simulink library "PrachLib"  (R2022a)
settings: Solver=VariableStepAuto  StartTime=0.0  StopTime=10.0  RelTol=1e-3
values from neighbouring files (symbols this model uses):
  ConfigTable = [16 1 9,20,20,20,20,20,20,20,20,20 0 2 6 2 4 ... (first row only)    [ConfigIndexTable.m]
  NTxAnts = 4    [setup_prach_shortFormat.m]    (also in setup_prach_shortFormat_fftShift.m)
undefined symbols (not defined in the file or in its folder): AdvDSPBChannelOutDisplay, AdvDSPBDMemDisplay, display, dpoly, dspba, dspba_ChannelInVis, dspba_ChannelOutVis, dspba_internal_get_channel_ports, evalAionMaskParam, InstanceNumber, latency, PRACH_regs, prach_short, primtype, UseDontCare, value
libraries: DSPBAPrim x280, DSPBAModelBus x7, DSPBAControl x7, $bdroot x3, DspbAdvFftLibrary x1, DSPBAVectorUtil x1
(part 3 of 4)

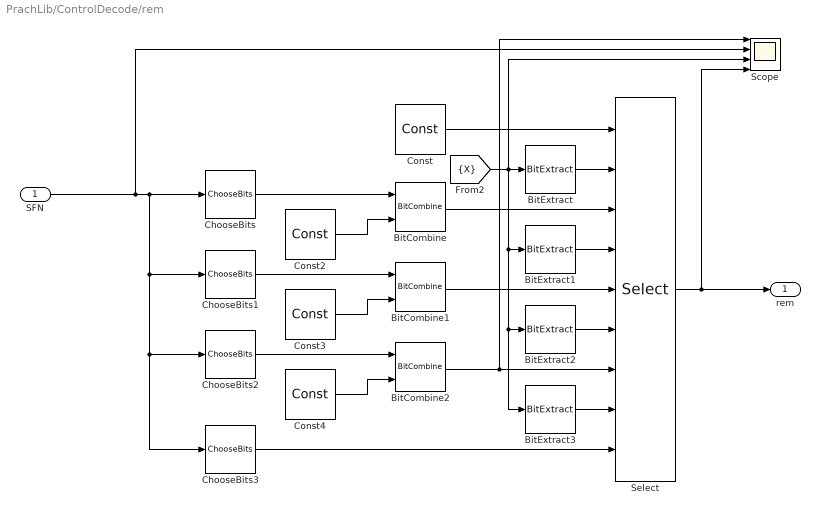
== system PrachLib/ControlDecode/rem ==
  SFN : Inport
  BitCombine : DSPBAPrim/BitCombine  primtype=bitcombine  nInputs=2  nOutputs=1  omode=Inherit via internal rule  otype=sfix(16)  scale=2^-15  rndmethod=Unbiased  factor=1  satmethod=Symmetric  shift_vec=[0 1 2 -1]  value=0  inPortNames=['l'; 'h';]  outPortNames=[' ']  dspbaimage=dspba_prim.svg  text=fprintf('[h,l]');  style=Optimised  visibilities=8+2  version=20211007
  BitCombine1 : DSPBAPrim/BitCombine  primtype=bitcombine  nInputs=2  nOutputs=1  omode=Inherit via internal rule  otype=sfix(16)  scale=2^-15  rndmethod=Unbiased  factor=1  satmethod=Symmetric  shift_vec=[0 1 2 -1]  value=0  inPortNames=['l'; 'h';]  outPortNames=[' ']  dspbaimage=dspba_prim.svg  text=fprintf('[h,l]');  style=Optimised  visibilities=8+2  version=20211007
  BitCombine2 : DSPBAPrim/BitCombine  primtype=bitcombine  nInputs=2  nOutputs=1  omode=Inherit via internal rule  otype=sfix(16)  scale=2^-15  rndmethod=Unbiased  factor=1  satmethod=Symmetric  shift_vec=[0 1 2 -1]  value=0  inPortNames=['l'; 'h';]  outPortNames=[' ']  dspbaimage=dspba_prim.svg  text=fprintf('[h,l]');  style=Optimised  visibilities=8+2  version=20211007
  BitExtract : DSPBAPrim/BitExtract  primtype=bitextract  nInputs=1  nOutputs=1  omode=boolean  otype=ufix(1)  scale=1  rndmethod=Unbiased  factor=1  satmethod=Symmetric  shift_vec=[0 1 2 -1]  value=1  inPortNames=[' '; ' ';]  outPortNames=[' ']  dspbaimage=dspba_prim.svg  text=fprintf('..%d', value);  style=Optimised  visibilities=8+1024  version=20211007
  BitExtract1 : DSPBAPrim/BitExtract  primtype=bitextract  nInputs=1  nOutputs=1  omode=boolean  otype=ufix(1)  scale=1  rndmethod=Unbiased  factor=1  satmethod=Symmetric  shift_vec=[0 1 2 -1]  value=2  inPortNames=[' '; ' ';]  outPortNames=[' ']  dspbaimage=dspba_prim.svg  text=fprintf('..%d', value);  style=Optimised  visibilities=8+1024  version=20211007
  BitExtract2 : DSPBAPrim/BitExtract  primtype=bitextract  nInputs=1  nOutputs=1  omode=boolean  otype=ufix(1)  scale=1  rndmethod=Unbiased  factor=1  satmethod=Symmetric  shift_vec=[0 1 2 -1]  value=3  inPortNames=[' '; ' ';]  outPortNames=[' ']  dspbaimage=dspba_prim.svg  text=fprintf('..%d', value);  style=Optimised  visibilities=8+1024  version=20211007
  BitExtract3 : DSPBAPrim/BitExtract  primtype=bitextract  nInputs=1  nOutputs=1  omode=boolean  otype=ufix(1)  scale=1  rndmethod=Unbiased  factor=1  satmethod=Symmetric  shift_vec=[0 1 2 -1]  value=4  inPortNames=[' '; ' ';]  outPortNames=[' ']  dspbaimage=dspba_prim.svg  text=fprintf('..%d', value);  style=Optimised  visibilities=8+1024  version=20211007
  ChooseBits : DSPBAPrim/ChooseBits  primtype=choosebits  nInputs=1  nOutputs=1  omode=Inherit via internal rule  otype=fixdt(0,1,1)  scale=1  rndmethod=Unbiased  factor=1  satmethod=Symmetric  shift_vec=[0 1 2 -1]  value=[0]  inPortNames=[' '; ' ';]  outPortNames=[' ']  dspbaimage=dspba_prim.svg  text=fprintf('%s',dspba.perm2str(value));  style=Optimised  visibilities=1024  version=20211007
  ChooseBits1 : DSPBAPrim/ChooseBits  primtype=choosebits  nInputs=1  nOutputs=1  omode=Inherit via internal rule  otype=fixdt(0,1,1)  scale=1  rndmethod=Unbiased  factor=1  satmethod=Symmetric  shift_vec=[0 1 2 -1]  value=[0,1]  inPortNames=[' '; ' ';]  outPortNames=[' ']  dspbaimage=dspba_prim.svg  text=fprintf('%s',dspba.perm2str(value));  style=Optimised  visibilities=1024  version=20211007
  ChooseBits2 : DSPBAPrim/ChooseBits  primtype=choosebits  nInputs=1  nOutputs=1  omode=Inherit via internal rule  otype=fixdt(0,1,1)  scale=1  rndmethod=Unbiased  factor=1  satmethod=Symmetric  shift_vec=[0 1 2 -1]  value=[0,1,2]  inPortNames=[' '; ' ';]  outPortNames=[' ']  dspbaimage=dspba_prim.svg  text=fprintf('%s',dspba.perm2str(value));  style=Optimised  visibilities=1024  version=20211007
  ChooseBits3 : DSPBAPrim/ChooseBits  primtype=choosebits  nInputs=1  nOutputs=1  omode=Inherit via internal rule  otype=fixdt(0,1,1)  scale=1  rndmethod=Unbiased  factor=1  satmethod=Symmetric  shift_vec=[0 1 2 -1]  value=[0,1,2,3]  inPortNames=[' '; ' ';]  outPortNames=[' ']  dspbaimage=dspba_prim.svg  text=fprintf('%s',dspba.perm2str(value));  style=Optimised  visibilities=1024  version=20211007
  Const : DSPBAPrim/Const  primtype=const  nInputs=0  nOutputs=1  omode=Specify via dialog  otype=ufix(4)  scale=1  rndmethod=Unbiased  factor=1  satmethod=Symmetric  shift_vec=[0 1 2 -1]  value=0  inPortNames=['+'; '+';]  outPortNames=[' ']  dspbaimage=dspba_prim.svg  text=fprintf('%s', num2str(value));  style=Optimised  visibilities=8 + 1024  floatPrecision=float32_m23  warnSaturation=on  version=20211007  SampleTime=inf
  Const2 : DSPBAPrim/Const  primtype=const  nInputs=0  nOutputs=1  omode=Specify via dialog  otype=ufix(3)  scale=1  rndmethod=Unbiased  factor=1  satmethod=Symmetric  shift_vec=[0 1 2 -1]  value=0  inPortNames=['+'; '+';]  outPortNames=[' ']  dspbaimage=dspba_prim.svg  text=fprintf('%s', num2str(value));  style=Optimised  visibilities=8 + 1024  floatPrecision=float32_m23  warnSaturation=on  version=20211007  SampleTime=inf
  Const3 : DSPBAPrim/Const  primtype=const  nInputs=0  nOutputs=1  omode=Specify via dialog  otype=ufix(2)  scale=1  rndmethod=Unbiased  factor=1  satmethod=Symmetric  shift_vec=[0 1 2 -1]  value=0  inPortNames=['+'; '+';]  outPortNames=[' ']  dspbaimage=dspba_prim.svg  text=fprintf('%s', num2str(value));  style=Optimised  visibilities=8 + 1024  floatPrecision=float32_m23  warnSaturation=on  version=20211007  SampleTime=inf
  Const4 : DSPBAPrim/Const  primtype=const  nInputs=0  nOutputs=1  omode=Specify via dialog  otype=ufix(1)  scale=1  rndmethod=Unbiased  factor=1  satmethod=Symmetric  shift_vec=[0 1 2 -1]  value=0  inPortNames=['+'; '+';]  outPortNames=[' ']  dspbaimage=dspba_prim.svg  text=fprintf('%s', num2str(value));  style=Optimised  visibilities=8 + 1024  floatPrecision=float32_m23  warnSaturation=on  version=20211007  SampleTime=inf
  Scope : Scope  NumInputPorts=4
  Select : DSPBAPrim/Select  primtype=select  nInputs=str2num(get_param(gcb,'value'))*2+1  nOutputs=1  omode=Inherit via internal rule  otype=sfix(16)  scale=2^-15  rndmethod=Unbiased  factor=1  satmethod=Symmetric  shift_vec=[0 1 2 -1]  value=4  inPortNames=['d'; '0'; 'a'; '1'; 'b'; '2'; 'c'; '3'; 'd'; '4'; 'e'; '5'; 'f'; '6'; 'g'; '7'; 'h'; '8'; 'i'; '9'; 'j']  outPortNames=[' ']  dspbaimage=dspba_prim_tall.svg  text=fprintf('%s', primtype);  style=Optimised  visibilities=8 + 1024  version=20211007
  rem : Outport
  wires:
  BitCombine2/1 -> Select/7, Scope/1
  SFN/1 -> ChooseBits/1, ChooseBits1/1, ChooseBits2/1, ChooseBits3/1, Scope/2
  [X] -> BitExtract/1, BitExtract3/1, BitExtract2/1, BitExtract1/1, Scope/3
  ChooseBits1/1 -> BitCombine1/1
  ChooseBits2/1 -> BitCombine2/1
  BitExtract1/1 -> Select/4
  ChooseBits/1 -> BitCombine/1
  BitCombine/1 -> Select/3
  Const2/1 -> BitCombine/2
  Const3/1 -> BitCombine1/2
  BitExtract/1 -> Select/2
  BitExtract3/1 -> Select/8
  Select/1 -> rem/1, Scope/4
  BitCombine1/1 -> Select/5
  Const4/1 -> BitCombine2/2
  BitExtract2/1 -> Select/6
  ChooseBits3/1 -> Select/9
  Const/1 -> Select/1

== system PrachLib/PRACH_CC/ScaleAndSelect ==
  vin : Inport
  chin : Inport  Port=2
  FFTSize : Inport  Port=3
  d : Inport  Port=4
  BWby10 : Inport  Port=5
  And1 : DSPBAPrim/And  primtype=and  nInputs=2  nOutputs=1  omode=Inherit via internal rule  otype=sfix(16)  scale=2^-15  rndmethod=Unbiased  factor=1  satmethod=Symmetric  shift_vec=[0 1 2 -1]  value=0  inPortNames=[' '; ' '; ' '; ' '; ' '; ' '; ' '; ' '; ' '; ' '; ' '; ' '; ' '; ' '; ' '; ' '; ]  outPortNames=[' ']  dspbaimage=dspba_prim.svg  text=fprintf('&');  style=Optimised  visibilities=8+2  version=20211007
  ChannelIn : DSPBAPrim/ChannelIn  primtype=channelin  nInputs=dspba_internal_get_channel_ports(gcb)  nOutputs=dspba_internal_get_channel_ports(gcb)  omode=Inherit via internal rule  otype=sfix(16)  scale=2^-15  rndmethod=Unbiased  factor=1  satmethod=Symmetric  shift_vec=[0 1 2 -1]  value=3  inPortNames=['v'; 'c'; '0'; '1'; '2'; '3'; '4'; '5'; '6'; '7'; '8'; '9'; 'A'; 'B'; 'D'; 'E'; 'F'; 'G'; 'H'; 'I'; 'J'; 'K'; 'L'; 'M'; 'N'; 'O'; 'P'; 'Q'; 'R'; 'S'; 'T'; 'U'; 'W'; 'X'; 'Y'; 'Z']  outPortNames=['v'; 'c'; '0'; '1'; '2'; '3'; '4'; '5'; '6'; '7'; '8'; '9'; 'A'; 'B'; 'D'; 'E'; 'F'; 'G'; 'H'; 'I'; 'J'; 'K'; 'L'; 'M'; 'N'; 'O'; 'P'; 'Q'; 'R'; 'S'; 'T'; 'U'; 'W'; 'X'; 'Y'; 'Z']  dspbaimage=dspba_prim_channel_tall.svg  text=fprintf('In');  style=Optimised  dataSignals=3  foldingEnabled=off  channels=1  sampleRate=200  packetBeginPresent=off  packetBeginEnabled=off  visibilities=dspba_ChannelInVis(gcb)  latencyCorrection=0  scheduleOrigin=off  version=20211214
  ChannelOut : DSPBAPrim/ChannelOut  primtype=channelout  nInputs=dspba_internal_get_channel_ports(gcb)  nOutputs=dspba_internal_get_channel_ports(gcb)  omode=Inherit via internal rule  otype=sfix(16)  scale=2^-15  rndmethod=Unbiased  factor=1  satmethod=Symmetric  shift_vec=[0 1 2 -1]  value=3  inPortNames=['v'; 'c'; '0'; '1'; '2'; '3'; '4'; '5'; '6'; '7'; '8'; '9'; 'A'; 'B'; 'D'; 'E'; 'F'; 'G'; 'H'; 'I'; 'J'; 'K'; 'L'; 'M'; 'N'; 'O'; 'P'; 'Q'; 'R'; 'S'; 'T'; 'U'; 'W'; 'X'; 'Y'; 'Z']  outPortNames=['v'; 'c'; '0'; '1'; '2'; '3'; '4'; '5'; '6'; '7'; '8'; '9'; 'A'; 'B'; 'D'; 'E'; 'F'; 'G'; 'H'; 'I'; 'J'; 'K'; 'L'; 'M'; 'N'; 'O'; 'P'; 'Q'; 'R'; 'S'; 'T'; 'U'; 'W'; 'X'; 'Y'; 'Z']  dspbaimage=dspba_prim_channel_tall.svg  text=fprintf('Out%s', AdvDSPBChannelOutDisplay(latency));  style=Optimised  dataSignals=3  foldingEnabled=off  channels=1  sampleRate=200  packetBeginPresent=off  packetBeginEnabled=off  visibilities=dspba_ChannelOutVis(gcb)  latency=0  latencyCorrection=0  version=20211214
  IndexCounter : Subsystem
  ScaleOutputAndCheck : Subsystem
      mask Display:
      | color('w');image('dspba_prim.jpg');
      | fprintf('*2^PRACH_fft_scale');
      | port_label('input',1,'din');
      | port_label('output',1,'dout');
  Sub : DSPBAPrim/Sub  primtype=sub  nInputs=2  nOutputs=1  omode=Inherit via internal rule with word growth  otype=sfix(16)  scale=2^-15  rndmethod=Unbiased  factor=1  satmethod=Symmetric  shift_vec=[0 1 2 -1]  value=0  inPortNames=['+'; '-';]  outPortNames=[' ']  dspbaimage=dspba_prim.svg  text=fprintf('-');  style=Optimised  visibilities=8+2^17+2^18  floatRounding=correct  advOptions=[]  version=20211007
  SynthesisInfo : DSPBAPrim/SynthesisInfo  primtype=synthinfo  nInputs=0  nOutputs=0  omode=Inherit via internal rule  otype=sfix(16)  scale=2^-15  rndmethod=Truncate  factor=1  satmethod=Symmetric  shift_vec=[0 1 2 -1]  value=99  inPortNames=[' '; ' ';]  outPortNames=[' ']  dspbaimage=dspba_prim_ctrl.jpg  text=fprintf('Style=%s', style);  style=Scheduled  visibilities=32768  constraintPair=None  constraintRelation=>  constraintLimit=6  modelRefSign=+  modelRef=''  showSchedule=off  simulationMode=Use Global Value  resetMinimization=Conditional - On for ChannelIn/Out only  version=20220106
  gen_139_valids : Subsystem
  qv : Outport  VectorParamsAs1DForOutWhenUnconnected=off
  qch : Outport  Port=2  VectorParamsAs1DForOutWhenUnconnected=off
  q : Outport  Port=3  VectorParamsAs1DForOutWhenUnconnected=off
  qv139 : Outport  Port=4  VectorParamsAs1DForOutWhenUnconnected=off
  FreqBinIdx : Outport  Port=5  VectorParamsAs1DForOutWhenUnconnected=off
  wires:
  ChannelOut/1 -> qv/1
  ChannelOut/2 -> qch/1
  ChannelIn/1 -> And1/1, ChannelOut/1, IndexCounter/1(v)
  ChannelIn/2 -> ChannelOut/2
  vin/1 -> ChannelIn/1
  chin/1 -> ChannelIn/2
  ChannelOut/3 -> q/1
  ChannelOut/4 -> qv139/1
  FFTSize/1 -> ChannelIn/3
  d/1 -> ChannelIn/4
  ChannelIn/4 -> ScaleOutputAndCheck/1(din)
  ChannelOut/5 -> FreqBinIdx/1
  BWby10/1 -> ChannelIn/5
  And1/1 -> ChannelOut/4
  IndexCounter/1(index) -> Sub/1, gen_139_valids/1(Index)
  gen_139_valids/1(v139) -> And1/2
  ChannelIn/5 -> gen_139_valids/3(BWby10)
  ChannelIn/3 -> gen_139_valids/2(FFTSize), IndexCounter/2(FFTSize)
  gen_139_valids/2(startSymFD) -> Sub/2
  Sub/1 -> ChannelOut/5
  ScaleOutputAndCheck/1(dout) -> ChannelOut/3

== system PrachLib/PRACH_CC/VFFT ==
  note: Bit-accurate simulation used
  note: Each block of 2^N samples should use the same channel
      | and starts arriving on the output after 2^N-1 cycles.
      |
      | So we latch the channel number and size on
      |  the last valid input of each block.
  v : Inport
  c : Inport  Port=2
  size : Inport  Port=3
  d : Inport  Port=4
  BWby10 : Inport  Port=5
  ChannelIn : DSPBAPrim/ChannelIn  primtype=channelin  nInputs=dspba_internal_get_channel_ports(gcb)  nOutputs=dspba_internal_get_channel_ports(gcb)  omode=Inherit via internal rule  otype=sfix(16)  scale=2^-15  rndmethod=Unbiased  factor=1  satmethod=Symmetric  shift_vec=[0 1 2 -1]  value=3  inPortNames=['v'; 'c'; '0'; '1'; '2'; '3'; '4'; '5'; '6'; '7'; '8'; '9'; 'a'; 'b']  outPortNames=['v'; 'c'; '0'; '1'; '2'; '3'; '4'; '5'; '6'; '7'; '8'; '9'; 'a'; 'b']  dspbaimage=dspba_prim_channel_tall.svg  text=fprintf('In');  style=Optimised  dataSignals=3  foldingEnabled=off  channels=1  sampleRate=200  packetBeginPresent=off  packetBeginEnabled=off  visibilities=dspba_ChannelInVis(gcb)  latencyCorrection=0  scheduleOrigin=on  version=20211214
  ChannelOut1 : DSPBAPrim/ChannelOut  primtype=channelout  nInputs=dspba_internal_get_channel_ports(gcb)  nOutputs=dspba_internal_get_channel_ports(gcb)  omode=Inherit via internal rule  otype=sfix(16)  scale=2^-15  rndmethod=Unbiased  factor=1  satmethod=Symmetric  shift_vec=[0 1 2 -1]  value=3  inPortNames=['v'; 'c'; '0'; '1'; '2'; '3'; '4'; '5'; '6'; '7'; '8'; '9']  outPortNames=['v'; 'c'; '0'; '1'; '2'; '3'; '4'; '5'; '6'; '7'; '8'; '9']  dspbaimage=dspba_prim_channel_tall.svg  text=fprintf('Out');  style=Optimised  dataSignals=3  foldingEnabled=off  channels=1  sampleRate=200  packetBeginPresent=off  packetBeginEnabled=off  visibilities=dspba_ChannelOutVis(gcb)  latency=0  latencyCorrection=0  version=20211214
  SynthesisInfo : DSPBAPrim/SynthesisInfo  primtype=synthinfo  nInputs=0  nOutputs=0  omode=Inherit via internal rule  otype=sfix(16)  scale=2^-15  rndmethod=Truncate  factor=1  satmethod=Symmetric  shift_vec=[0 1 2 -1]  value=99  inPortNames=[' '; ' ';]  outPortNames=[' ']  dspbaimage=dspba_prim_ctrl.jpg  text=fprintf('Style=%s', style);  style=Scheduled  visibilities=32768  constraintPair=None  constraintRelation=>  constraintLimit=2  modelRefSign=+  modelRef=''  showSchedule=off  simulationMode=Bit Accurate  resetMinimization=Conditional - On for ChannelIn/Out only  version=20220106
  VFFT_Light : DspbAdvFftLibrary/Common/VFFT_Light  IFFT=IFFT  subchannels=subchannels  br_in=br_in  maxSize=maxSize  minSize=minSize  in_type=in_type  type_strings=type_strings  faithful=faithful  wirecount=1
  latch_0L : DSPBAControl/latch_0L
  latch_0L1 : DSPBAControl/latch_0L
  latch_0L2 : DSPBAControl/latch_0L
  qv : Outport
  qc : Outport  Port=2
  qsize : Outport  Port=3
  q : Outport  Port=4
  qBWby10 : Outport  Port=5
  wires:
  VFFT_Light/2 -> ChannelOut1/4
  latch_0L1/1 -> ChannelOut1/3
  ChannelOut1/3 -> qsize/1
  ChannelOut1/4 -> q/1
  ChannelIn/4 -> VFFT_Light/3
  ChannelIn/3 -> VFFT_Light/2, latch_0L1/2
  d/1 -> ChannelIn/4
  size/1 -> ChannelIn/3
  v/1 -> ChannelIn/1
  c/1 -> ChannelIn/2
  latch_0L/1 -> ChannelOut1/2
  ChannelIn/2 -> latch_0L/2
  ChannelOut1/1 -> qv/1
  ChannelOut1/2 -> qc/1
  VFFT_Light/1 -> ChannelOut1/1
  ChannelIn/1 -> VFFT_Light/1
  VFFT_Light/3 -> latch_0L2/1, latch_0L1/1, latch_0L/1
  BWby10/1 -> ChannelIn/5
  ChannelIn/5 -> latch_0L2/2
  latch_0L2/1 -> ChannelOut1/5
  ChannelOut1/5 -> qBWby10/1

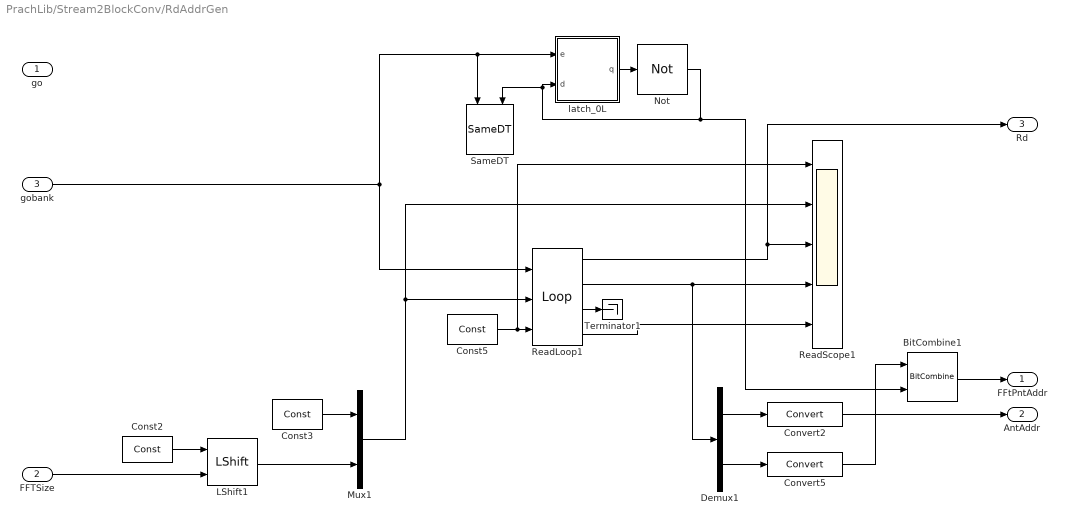
== system PrachLib/Stream2BlockConv/RdAddrGen ==
  go : Inport
  FFTSize : Inport  Port=2
  gobank : Inport  Port=3
  BitCombine1 : DSPBAPrim/BitCombine  primtype=bitcombine  nInputs=2  nOutputs=1  omode=Inherit via internal rule  otype=sfix(16)  scale=2^-15  rndmethod=Unbiased  factor=1  satmethod=Symmetric  shift_vec=[0 1 2 -1]  value=0  inPortNames=['l'; 'h';]  outPortNames=[' ']  dspbaimage=dspba_prim.svg  text=fprintf('[h,l]');  style=Optimised  visibilities=8+2  version=20211007
  Const2 : DSPBAPrim/Const  primtype=const  nInputs=0  nOutputs=1  omode=Inherit via internal rule  otype=sfix(16)  scale=2^-15  rndmethod=Unbiased  factor=1  satmethod=Symmetric  shift_vec=[0 1 2 -1]  value=1  inPortNames=['+'; '+';]  outPortNames=[' ']  dspbaimage=dspba_prim.svg  text=fprintf('%s', num2str(value));  style=Optimised  visibilities=8 + 1024  floatPrecision=float32_m23  warnSaturation=on  version=20211007  SampleTime=inf
  Const3 : DSPBAPrim/Const  primtype=const  nInputs=0  nOutputs=1  omode=Inherit via back propagation  otype=sfix(16)  scale=2^-15  rndmethod=Unbiased  factor=1  satmethod=Symmetric  shift_vec=[0 1 2 -1]  value=NAnts  inPortNames=['+'; '+';]  outPortNames=[' ']  dspbaimage=dspba_prim.svg  text=fprintf('%s', num2str(value));  style=Optimised  visibilities=8 + 1024  floatPrecision=float32_m23  warnSaturation=on  version=20211007  SampleTime=inf
  Const5 : DSPBAPrim/Const  primtype=const  nInputs=0  nOutputs=1  omode=boolean  otype=sfix(16)  scale=2^-15  rndmethod=Unbiased  factor=1  satmethod=Symmetric  shift_vec=[0 1 2 -1]  value=1  inPortNames=['+'; '+';]  outPortNames=[' ']  dspbaimage=dspba_prim.svg  text=fprintf('%s', num2str(value));  style=Optimised  visibilities=8 + 1024  floatPrecision=float32_m23  warnSaturation=on  version=20211007  SampleTime=inf
  Convert2 : DSPBAPrim/Convert  primtype=convert  nInputs=1  nOutputs=1  omode=Specify via dialog  otype=ufix(ceil(log2(NAnts)))  scale=1  rndmethod=Truncate  factor=1  satmethod=None  shift_vec=[0 1 2 -1]  value=round([0:255]/17)  inPortNames=[' '; ' ';]  outPortNames=[' '; 'c']  dspbaimage=dspba_prim_wide.svg  text=fprintf('convert');  style=Optimised  visibilities=8+64+256+2^17  clipdetect=off  floatPrecision=float32_m23  advOptions=[]  version=20211007
  Convert5 : DSPBAPrim/Convert  primtype=convert  nInputs=1  nOutputs=1  omode=Specify via dialog  otype=ufix(ceil(log2(NFftMax)))  scale=1  rndmethod=Truncate  factor=1  satmethod=None  shift_vec=[0 1 2 -1]  value=round([0:255]/17)  inPortNames=[' '; ' ';]  outPortNames=[' '; 'c']  dspbaimage=dspba_prim_wide.svg  text=fprintf('convert');  style=Optimised  visibilities=8+64+256+2^17  clipdetect=off  floatPrecision=float32_m23  advOptions=[]  version=20211007
  Demux1 : Demux  Outputs=2
  LShift1 : DSPBAPrim/LShift  primtype=lshift  nInputs=2  nOutputs=1  omode=Specify via dialog  otype=ufix(log2(NFftMax)+1)  scale=1  rndmethod=Unbiased  factor=1  satmethod=Symmetric  shift_vec=[0 1 2 -1]  value=0  inPortNames=['a'; 'b';]  outPortNames=[' ']  dspbaimage=dspba_prim.svg  text=fprintf('a << b');  style=Optimised  visibilities=8  version=20211007
  Mux1 : Mux  Inputs=2
  Not : DSPBAPrim/Not  primtype=not  nInputs=1  nOutputs=1  omode=Inherit via internal rule  otype=sfix(16)  scale=2^-15  rndmethod=Unbiased  factor=1  satmethod=Symmetric  shift_vec=[0 1 2 -1]  value=0  inPortNames=[' '; ' ';]  outPortNames=[' ']  dspbaimage=dspba_prim.svg  text=fprintf('~');  style=Optimised  visibilities=8  version=20211007
  ReadLoop1 : DSPBAPrim/Loop  primtype=loop  nInputs=3  nOutputs=4  omode=Inherit via internal rule  otype=sfix(16)  scale=2^-15  rndmethod=Unbiased  factor=1  satmethod=Symmetric  shift_vec=[0 1 2 -1]  value=[zeros(16, 1)]  inPortNames=['g'; 'c'; 'e']  outPortNames=['v'; 'q'; 'f'; 'l']  dspbaimage=dspba_prim_tall.svg  text=fprintf('loop');  style=Optimised  visibilities=0  version=20211007
  ReadScope1 : Scope  NumInputPorts=5
  SameDT : DSPBAControl/SameDT
  Terminator1 : Terminator
  latch_0L : Subsystem  AncestorBlock=DSPBAControl/latch_0L
      mask help: The latch_0 block enable signal has an immediate effect on the output. While the enable is high,the data passes straight through.When the enable goes low, the latch_0 block outputs and holds the data input from the previous cycle.
      mask Help: helpview(dspba.GetHelp('latch_0L'));
      mask Display:
      | color('w');
      | image('dspba_prim_masked.png');
      | fprintf('0L\nlatch');
      | port_label('input',1,'e');
      | port_label('input',2,'d');
      | port_label('output',1,'q');
  FFtPntAddr : Outport
  AntAddr : Outport  Port=2
  Rd : Outport  Port=3
  wires:
  latch_0L/1(q) -> Not/1
  BitCombine1/1 -> FFtPntAddr/1
  gobank/1 -> ReadLoop1/1, latch_0L/1(e), SameDT/1
  Not/1 -> BitCombine1/2, SameDT/2, latch_0L/2(d)
  Demux1/2 -> Convert5/1
  Demux1/1 -> Convert2/1
  Const2/1 -> LShift1/1
  Mux1/1 -> ReadLoop1/2, ReadScope1/2
  Const5/1 -> ReadScope1/1, ReadLoop1/3
  FFTSize/1 -> LShift1/2
  ReadLoop1/2 -> Demux1/1, ReadScope1/4
  ReadLoop1/1 -> ReadScope1/3, Rd/1
  Const3/1 -> Mux1/1
  ReadLoop1/3 -> Terminator1/1
  Convert5/1 -> BitCombine1/1
  LShift1/1 -> Mux1/2
  ReadLoop1/4 -> ReadScope1/5
  Convert2/1 -> AntAddr/1

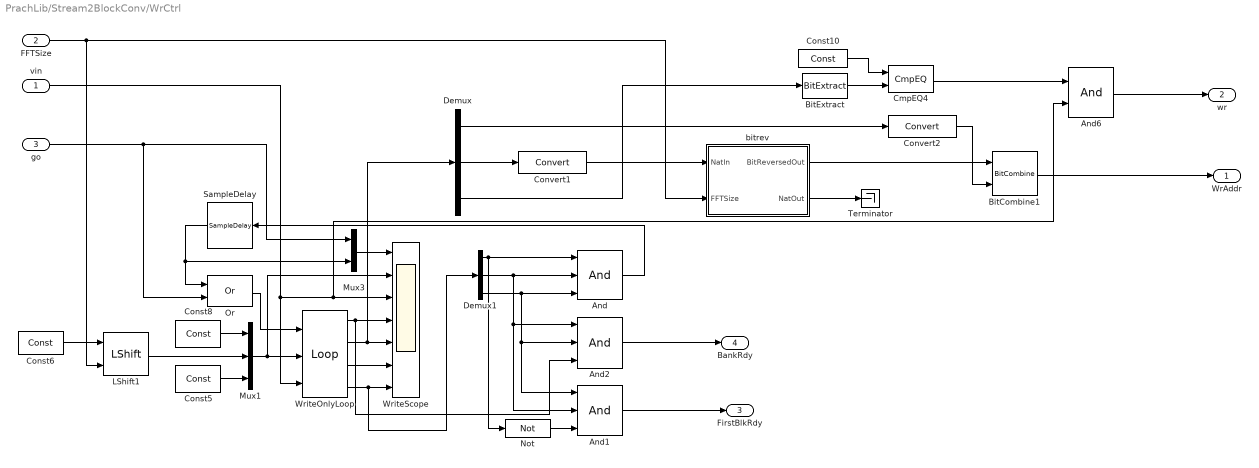
== system PrachLib/Stream2BlockConv/WrCtrl ==
  vin : Inport
  FFTSize : Inport  Port=2
  go : Inport  Port=3
  And : DSPBAPrim/And  primtype=and  nInputs=3  nOutputs=1  omode=Inherit via internal rule  otype=sfix(16)  scale=2^-15  rndmethod=Unbiased  factor=1  satmethod=Symmetric  shift_vec=[0 1 2 -1]  value=0  inPortNames=[' '; ' '; ' '; ' '; ' '; ' '; ' '; ' '; ' '; ' '; ' '; ' '; ' '; ' '; ' '; ' '; ]  outPortNames=[' ']  dspbaimage=dspba_prim.svg  text=fprintf('&');  style=Optimised  visibilities=8+2  version=20211007
  And1 : DSPBAPrim/And  primtype=and  nInputs=3  nOutputs=1  omode=Inherit via internal rule  otype=sfix(16)  scale=2^-15  rndmethod=Unbiased  factor=1  satmethod=Symmetric  shift_vec=[0 1 2 -1]  value=0  inPortNames=[' '; ' '; ' '; ' '; ' '; ' '; ' '; ' '; ' '; ' '; ' '; ' '; ' '; ' '; ' '; ' '; ]  outPortNames=[' ']  dspbaimage=dspba_prim.svg  text=fprintf('&');  style=Optimised  visibilities=8+2  version=20211007
  And2 : DSPBAPrim/And  primtype=and  nInputs=3  nOutputs=1  omode=Inherit via internal rule  otype=sfix(16)  scale=2^-15  rndmethod=Unbiased  factor=1  satmethod=Symmetric  shift_vec=[0 1 2 -1]  value=0  inPortNames=[' '; ' '; ' '; ' '; ' '; ' '; ' '; ' '; ' '; ' '; ' '; ' '; ' '; ' '; ' '; ' '; ]  outPortNames=[' ']  dspbaimage=dspba_prim.svg  text=fprintf('&');  style=Optimised  visibilities=8+2  version=20211007
  And6 : DSPBAPrim/And  primtype=and  nInputs=2  nOutputs=1  omode=Inherit via internal rule  otype=sfix(16)  scale=2^-15  rndmethod=Unbiased  factor=1  satmethod=Symmetric  shift_vec=[0 1 2 -1]  value=0  inPortNames=[' '; ' '; ' '; ' '; ' '; ' '; ' '; ' '; ' '; ' '; ' '; ' '; ' '; ' '; ' '; ' '; ]  outPortNames=[' ']  dspbaimage=dspba_prim.svg  text=fprintf('&');  style=Optimised  visibilities=8+2  version=20211007
  BitCombine1 : DSPBAPrim/BitCombine  primtype=bitcombine  nInputs=2  nOutputs=1  omode=Inherit via internal rule  otype=sfix(16)  scale=2^-15  rndmethod=Unbiased  factor=1  satmethod=Symmetric  shift_vec=[0 1 2 -1]  value=0  inPortNames=['l'; 'h';]  outPortNames=[' ']  dspbaimage=dspba_prim.svg  text=fprintf('[h,l]');  style=Optimised  visibilities=8+2  version=20211007
  BitExtract : DSPBAPrim/BitExtract  primtype=bitextract  nInputs=1  nOutputs=1  omode=Specify via dialog  otype=ufix(ceil(log2(NTxAnts)))  scale=1  rndmethod=Unbiased  factor=1  satmethod=Symmetric  shift_vec=[0 1 2 -1]  value=0  inPortNames=[' '; ' ';]  outPortNames=[' ']  dspbaimage=dspba_prim.svg  text=fprintf('..%d', value);  style=Optimised  visibilities=8+1024  version=20211007
  CmpEQ4 : DSPBAPrim/CmpEQ  primtype=cmpeq  nInputs=2  nOutputs=1  omode=boolean  otype=sfix(16)  scale=2^-15  rndmethod=Unbiased  factor=1  satmethod=Symmetric  shift_vec=[0 1 2 -1]  value=0  inPortNames=[' '; ' ';]  outPortNames=[' ']  dspbaimage=dspba_prim.svg  text=fprintf('==');  style=Optimised  visibilities=0  advOptions=[]  version=20211007
  Const10 : DSPBAPrim/Const  primtype=const  nInputs=0  nOutputs=1  omode=Inherit via internal rule  otype=sfix(16)  scale=2^-15  rndmethod=Unbiased  factor=1  satmethod=Symmetric  shift_vec=[0 1 2 -1]  value=0:(NTxAnts-1)  inPortNames=['+'; '+';]  outPortNames=[' ']  dspbaimage=dspba_prim.svg  text=fprintf('%s', num2str(value));  style=Optimised  visibilities=8 + 1024  floatPrecision=float32_m23  warnSaturation=on  version=20211007  SampleTime=inf
  Const5 : DSPBAPrim/Const  primtype=const  nInputs=0  nOutputs=1  omode=Inherit via back propagation  otype=sfix(16)  scale=2^-15  rndmethod=Unbiased  factor=1  satmethod=Symmetric  shift_vec=[0 1 2 -1]  value=NAnts  inPortNames=['+'; '+';]  outPortNames=[' ']  dspbaimage=dspba_prim.svg  text=fprintf('%s', num2str(value));  style=Optimised  visibilities=8 + 1024  floatPrecision=float32_m23  warnSaturation=on  version=20211007  SampleTime=inf
  Const6 : DSPBAPrim/Const  primtype=const  nInputs=0  nOutputs=1  omode=Inherit via internal rule  otype=sfix(16)  scale=2^-15  rndmethod=Unbiased  factor=1  satmethod=Symmetric  shift_vec=[0 1 2 -1]  value=1  inPortNames=['+'; '+';]  outPortNames=[' ']  dspbaimage=dspba_prim.svg  text=fprintf('%s', num2str(value));  style=Optimised  visibilities=8 + 1024  floatPrecision=float32_m23  warnSaturation=on  version=20211007  SampleTime=inf
  Const8 : DSPBAPrim/Const  primtype=const  nInputs=0  nOutputs=1  omode=Inherit via back propagation  otype=sfix(16)  scale=2^-15  rndmethod=Unbiased  factor=1  satmethod=Symmetric  shift_vec=[0 1 2 -1]  value=2  inPortNames=['+'; '+';]  outPortNames=[' ']  dspbaimage=dspba_prim.svg  text=fprintf('%s', num2str(value));  style=Optimised  visibilities=8 + 1024  floatPrecision=float32_m23  warnSaturation=on  version=20211007  SampleTime=inf
  Convert1 : DSPBAPrim/Convert  primtype=convert  nInputs=1  nOutputs=1  omode=Specify via dialog  otype=ufix(ceil(log2(NFftMax)))  scale=1  rndmethod=Truncate  factor=1  satmethod=None  shift_vec=[0 1 2 -1]  value=round([0:255]/17)  inPortNames=[' '; ' ';]  outPortNames=[' '; 'c']  dspbaimage=dspba_prim_wide.svg  text=fprintf('convert');  style=Optimised  visibilities=8+64+256+2^17  clipdetect=off  floatPrecision=float32_m23  advOptions=[]  version=20211007
  Convert2 : DSPBAPrim/Convert  primtype=convert  nInputs=1  nOutputs=1  omode=Specify via dialog  otype=ufix(1)  scale=1  rndmethod=Truncate  factor=1  satmethod=None  shift_vec=[0 1 2 -1]  value=round([0:255]/17)  inPortNames=[' '; ' ';]  outPortNames=[' '; 'c']  dspbaimage=dspba_prim_wide.svg  text=fprintf('convert');  style=Optimised  visibilities=8+64+256+2^17  clipdetect=off  floatPrecision=float32_m23  advOptions=[]  version=20211007
  Demux : Demux  Outputs=3
  Demux1 : Demux  Outputs=3
  LShift1 : DSPBAPrim/LShift  primtype=lshift  nInputs=2  nOutputs=1  omode=Specify via dialog  otype=ufix(log2(NFftMax)+1)  scale=1  rndmethod=Unbiased  factor=1  satmethod=Symmetric  shift_vec=[0 1 2 -1]  value=0  inPortNames=['a'; 'b';]  outPortNames=[' ']  dspbaimage=dspba_prim.svg  text=fprintf('a << b');  style=Optimised  visibilities=8  version=20211007
  Mux1 : Mux  Inputs=3
  Mux3 : Mux  Inputs=2
  Not : DSPBAPrim/Not  primtype=not  nInputs=1  nOutputs=1  omode=Inherit via internal rule  otype=sfix(16)  scale=2^-15  rndmethod=Unbiased  factor=1  satmethod=Symmetric  shift_vec=[0 1 2 -1]  value=0  inPortNames=[' '; ' ';]  outPortNames=[' ']  dspbaimage=dspba_prim.svg  text=fprintf('~');  style=Optimised  visibilities=8  version=20211007
  Or : DSPBAPrim/Or  primtype=or  nInputs=2  nOutputs=1  omode=Inherit via internal rule  otype=sfix(16)  scale=2^-15  rndmethod=Unbiased  factor=1  satmethod=Symmetric  shift_vec=[0 1 2 -1]  value=0  inPortNames=[' '; ' '; ' '; ' '; ' '; ' '; ' '; ' '; ' '; ' '; ' '; ' '; ' '; ' '; ' '; ' '; ]  outPortNames=[' ']  dspbaimage=dspba_prim.svg  text=fprintf('|');  style=Optimised  visibilities=8+2  version=20211007
  SampleDelay : DSPBAPrim/SampleDelay  primtype=sampdelay  nInputs=1  nOutputs=1  omode=Inherit via internal rule  otype=sfix(16)  scale=2^-15  rndmethod=Unbiased  factor=1  satmethod=Symmetric  shift_vec=[0 1 2 -1]  floatPrecision=float32_m23  value=1  inPortNames=[' '; ' ';]  outPortNames=[' ']  dspbaimage=dspba_prim.svg  text=dpoly(1, eye(1,value+1), 'z')  style=Optimised  visibilities=8 + 1024 + 2^17 + 2^18  flexible=off  slackgroup=0  augmented=0  version=20211007  advOptions=[]
  Terminator : Terminator
  WriteOnlyLoop : DSPBAPrim/Loop  primtype=loop  nInputs=3  nOutputs=4  omode=Inherit via internal rule  otype=sfix(16)  scale=2^-15  rndmethod=Unbiased  factor=1  satmethod=Symmetric  shift_vec=[0 1 2 -1]  value=[zeros(16, 1)]  inPortNames=['g'; 'c'; 'e']  outPortNames=['v'; 'q'; 'f'; 'l']  dspbaimage=dspba_prim_tall.svg  text=fprintf('loop');  style=Optimised  visibilities=0  version=20211007
  WriteScope : Scope  NumInputPorts=7
  bitrev : Subsystem  mask{NFftMax=NFftMax}
      mask prompts: NFftMax "Maximum FFT size"
  WrAddr : Outport
  wr : Outport  Port=2
  FirstBlkRdy : Outport  Port=3
  BankRdy : Outport  Port=4
  wires:
  And2/1 -> BankRdy/1
  bitrev/1(BitReversedOut) -> BitCombine1/1
  bitrev/2(NatOut) -> Terminator/1
  And6/1 -> wr/1
  Convert2/1 -> BitCombine1/2
  Mux3/1 -> WriteScope/1
  Const10/1 -> CmpEQ4/1
  Convert1/1 -> bitrev/1(NatIn)
  And/1 -> SampleDelay/1
  LShift1/1 -> Mux1/2
  Const6/1 -> LShift1/1
  BitCombine1/1 -> WrAddr/1
  vin/1 -> WriteScope/3, And6/2, WriteOnlyLoop/3
  Demux1/3 -> And/3, And2/2, And1/1
  WriteOnlyLoop/4 -> Demux1/1, WriteScope/7
  And1/1 -> FirstBlkRdy/1
  FFTSize/1 -> bitrev/2(FFTSize), LShift1/2
  Or/1 -> WriteOnlyLoop/1
  WriteOnlyLoop/3 -> WriteScope/6
  SampleDelay/1 -> Mux3/2, Or/1
  Demux1/2 -> And/2, And2/1, And1/2
  Demux/3 -> BitExtract/1
  Demux/2 -> Convert1/1
  Demux1/1 -> Not/1, And/1
  Not/1 -> And1/3
  Demux/1 -> Convert2/1
  BitExtract/1 -> CmpEQ4/2
  Mux1/1 -> WriteScope/2, WriteOnlyLoop/2
  WriteOnlyLoop/1 -> WriteScope/4, And2/3
  WriteOnlyLoop/2 -> WriteScope/5, Demux/1
  Const5/1 -> Mux1/3
  go/1 -> Or/2, Mux3/1
  Const8/1 -> Mux1/1
  CmpEQ4/1 -> And6/1

== system PrachLib/PRACH_CC/ScaleAndSelect/IndexCounter ==
  v : Inport
  FFTSize : Inport  Port=2
  And : DSPBAPrim/And  primtype=and  nInputs=2  nOutputs=1  omode=Inherit via internal rule  otype=sfix(16)  scale=2^-15  rndmethod=Unbiased  factor=1  satmethod=Symmetric  shift_vec=[0 1 2 -1]  value=0  inPortNames=[' '; ' '; ' '; ' '; ' '; ' '; ' '; ' '; ' '; ' '; ' '; ' '; ' '; ' '; ' '; ' '; ]  outPortNames=[' ']  dspbaimage=dspba_prim.svg  text=fprintf('&');  style=Optimised  visibilities=8+2  version=20211007
  BitCombine1 : DSPBAPrim/BitCombine  primtype=bitcombine  nInputs=2  nOutputs=1  omode=Inherit via internal rule  otype=sfix(16)  scale=2^-15  rndmethod=Unbiased  factor=1  satmethod=Symmetric  shift_vec=[0 1 2 -1]  value=0  inPortNames=['l'; 'h';]  outPortNames=[' ']  dspbaimage=dspba_prim.svg  text=fprintf('[h,l]');  style=Optimised  visibilities=8+2  version=20211007
  BitExtract1 : DSPBAPrim/BitExtract  primtype=bitextract  nInputs=1  nOutputs=1  omode=Inherit via internal rule  otype=ufix(1)  scale=1  rndmethod=Unbiased  factor=1  satmethod=Symmetric  shift_vec=[0 1 2 -1]  value=1  inPortNames=[' '; ' ';]  outPortNames=[' ']  dspbaimage=dspba_prim.svg  text=fprintf('..%d', value);  style=Optimised  visibilities=8+1024  version=20211007
  Const : DSPBAPrim/Const  primtype=const  nInputs=0  nOutputs=1  omode=Inherit via internal rule  otype=sfix(16)  scale=2^-15  rndmethod=Unbiased  factor=1  satmethod=Symmetric  shift_vec=[0 1 2 -1]  value=1  inPortNames=['+'; '+';]  outPortNames=[' ']  dspbaimage=dspba_prim.svg  text=fprintf('%s', num2str(value));  style=Optimised  visibilities=8 + 1024  floatPrecision=float32_m23  warnSaturation=on  version=20211007  SampleTime=inf
  Const4 : DSPBAPrim/Const  primtype=const  nInputs=0  nOutputs=1  omode=Inherit via internal rule  otype=sfix(16)  scale=2^-15  rndmethod=Unbiased  factor=1  satmethod=Symmetric  shift_vec=[0 1 2 -1]  value=0  inPortNames=['+'; '+';]  outPortNames=[' ']  dspbaimage=dspba_prim.svg  text=fprintf('%s', num2str(value));  style=Optimised  visibilities=8 + 1024  floatPrecision=float32_m23  warnSaturation=on  version=20211007  SampleTime=inf
  LShift : DSPBAPrim/LShift  primtype=lshift  nInputs=2  nOutputs=1  omode=Specify via dialog  otype=ufix(log2(prach_short.Nfft)+1)  scale=1  rndmethod=Unbiased  factor=1  satmethod=Symmetric  shift_vec=[0 1 2 -1]  value=0  inPortNames=['a'; 'b';]  outPortNames=[' ']  dspbaimage=dspba_prim.svg  text=fprintf('a << b');  style=Optimised  visibilities=8  version=20211007
  Loop : DSPBAPrim/Loop  primtype=loop  nInputs=3  nOutputs=4  omode=Inherit via internal rule  otype=sfix(16)  scale=2^-15  rndmethod=Unbiased  factor=1  satmethod=Symmetric  shift_vec=[0 1 2 -1]  value=[zeros(16, 1)]  inPortNames=['g'; 'c'; 'e']  outPortNames=['v'; 'q'; 'f'; 'l']  dspbaimage=dspba_prim_tall.svg  text=fprintf('loop');  style=Optimised  visibilities=0  version=20211007
  Not : DSPBAPrim/Not  primtype=not  nInputs=1  nOutputs=1  omode=Inherit via internal rule  otype=sfix(16)  scale=2^-15  rndmethod=Unbiased  factor=1  satmethod=Symmetric  shift_vec=[0 1 2 -1]  value=0  inPortNames=[' '; ' ';]  outPortNames=[' ']  dspbaimage=dspba_prim.svg  text=fprintf('~');  style=Optimised  visibilities=8  version=20211007
  Or1 : DSPBAPrim/Or  primtype=or  nInputs=2  nOutputs=1  omode=Inherit via internal rule  otype=sfix(16)  scale=2^-15  rndmethod=Unbiased  factor=1  satmethod=Symmetric  shift_vec=[0 1 2 -1]  value=0  inPortNames=[' '; ' '; ' '; ' '; ' '; ' '; ' '; ' '; ' '; ' '; ' '; ' '; ' '; ' '; ' '; ' '; ]  outPortNames=[' ']  dspbaimage=dspba_prim.svg  text=fprintf('|');  style=Optimised  visibilities=8+2  version=20211007
  SampleDelay1 : DSPBAPrim/SampleDelay  primtype=sampdelay  nInputs=1  nOutputs=1  omode=Inherit via internal rule  otype=sfix(16)  scale=2^-15  rndmethod=Unbiased  factor=1  satmethod=Symmetric  shift_vec=[0 1 2 -1]  floatPrecision=float32_m23  value=1  inPortNames=[' '; ' ';]  outPortNames=[' ']  dspbaimage=dspba_prim.svg  text=dpoly(1, eye(1,value+1), 'z')  style=Optimised  visibilities=8 + 1024 + 2^17 + 2^18  flexible=off  slackgroup=0  augmented=0  version=20211007  advOptions=[]
  SampleDelay2 : DSPBAPrim/SampleDelay  primtype=sampdelay  nInputs=1  nOutputs=1  omode=Inherit via internal rule  otype=sfix(16)  scale=2^-15  rndmethod=Unbiased  factor=1  satmethod=Symmetric  shift_vec=[0 1 2 -1]  floatPrecision=float32_m23  value=1  inPortNames=[' '; ' ';]  outPortNames=[' ']  dspbaimage=dspba_prim.svg  text=dpoly(1, eye(1,value+1), 'z')  style=Optimised  visibilities=8 + 1024 + 2^17 + 2^18  flexible=off  slackgroup=0  augmented=0  version=20211007  advOptions=[]
  Scope2 : Scope  NumInputPorts=7
  Terminator : Terminator
  Terminator1 : Terminator
  Xor3 : DSPBAPrim/Xor  primtype=xor  nInputs=2  nOutputs=1  omode=Inherit via internal rule  otype=sfix(16)  scale=2^-15  rndmethod=Unbiased  factor=1  satmethod=Symmetric  shift_vec=[0 1 2 -1]  value=0  inPortNames=[' '; ' '; ' '; ' '; ' '; ' '; ' '; ' '; ' '; ' '; ' '; ' '; ' '; ' '; ' '; ' '; ]  outPortNames=[' ']  dspbaimage=dspba_prim.svg  text=fprintf('^');  style=Optimised  visibilities=8+2  version=20211007
  index : Outport
  wires:
  Not/1 -> And/2
  SampleDelay1/1 -> Not/1
  Const/1 -> LShift/1
  FFTSize/1 -> LShift/2
  v/1 -> Loop/3, SampleDelay1/1, And/1
  Const4/1 -> BitCombine1/2
  LShift/1 -> BitExtract1/1, Scope2/2, Loop/2
  Loop/2 -> Scope2/1, Xor3/1
  Xor3/1 -> index/1, Scope2/3
  BitCombine1/1 -> Scope2/4, Xor3/2
  BitExtract1/1 -> BitCombine1/1, Scope2/5
  Or1/1 -> Scope2/6, Loop/1
  And/1 -> Or1/2, Scope2/7
  Loop/4 -> SampleDelay2/1
  SampleDelay2/1 -> Or1/1
  Loop/3 -> Terminator1/1
  Loop/1 -> Terminator/1

== system PrachLib/PRACH_CC/ScaleAndSelect/ScaleOutputAndCheck ==
  din : Inport
  Assertion : Assertion  AssertionFailFcn="display(' *** Clipping occurred in ScaleAndSelect block.  Please check the PRACH_fft_scale register value')"
  RegField2 : DSPBAModelBus/RegField  reg_name=PRACH_regs(InstanceNumber).PRACH_fft_scale_addr  reg_rwmode=Read/Write  reg_msb=7  reg_lsb=0  reg_mode=Specify via dialog  reg_type=uint(8)  reg_scale=2^0  reg_init=PRACH_regs(InstanceNumber).PRACH_fft_scale  reg_desc=PRACH_regs(InstanceNumber).PRACH_fft_scale_string  reg_modal=off  reg_desc0=0  reg_desc1=0  reg_desc2=0  reg_desc3=0  reg_desc4=0  reg_desc5=0  reg_desc6=0  reg_desc7=0  reg_addr=12  SampleTime=-1  version=20090407
  Relational Operator : RelationalOperator  Operator===  OutDataTypeStr=boolean  RndMeth=Simplest  InputSameDT=off
  SampleDelay1 : DSPBAPrim/SampleDelay  primtype=sampdelay  nInputs=1  nOutputs=1  omode=Inherit via internal rule  otype=sfix(16)  scale=2^-15  rndmethod=Unbiased  factor=1  satmethod=Symmetric  shift_vec=[0 1 2 -1]  floatPrecision=float32_m23  value=1  inPortNames=[' '; ' ';]  outPortNames=[' ']  dspbaimage=dspba_prim.svg  text=dpoly(1, eye(1,value+1), 'z')  style=Optimised  visibilities=8 + 1024 + 2^17 + 2^18  flexible=off  slackgroup=0  augmented=0  version=20211007  advOptions=[]
  SampleDelay2 : DSPBAPrim/SampleDelay  primtype=sampdelay  nInputs=1  nOutputs=1  omode=Inherit via internal rule  otype=sfix(16)  scale=2^-15  rndmethod=Unbiased  factor=1  satmethod=Symmetric  shift_vec=[0 1 2 -1]  floatPrecision=float32_m23  value=1  inPortNames=[' '; ' ';]  outPortNames=[' ']  dspbaimage=dspba_prim.svg  text=dpoly(1, eye(1,value+1), 'z')  style=Optimised  visibilities=8 + 1024 + 2^17 + 2^18  flexible=off  slackgroup=0  augmented=0  version=20211007  advOptions=[]
  Scope : Scope  Commented=on  NumInputPorts=4
  Shift : DSPBAPrim/Shift  primtype=shift  nInputs=2  nOutputs=1  omode=Specify via dialog  otype=sfix(16)  scale=2^-15  rndmethod=Unbiased  factor=1  satmethod=Symmetric  shift_vec=[0 1 2 -1]  value=0  inPortNames=['a'; 'b';]  outPortNames=[' ']  dspbaimage=dspba_prim.svg  text=fprintf('a >> b');  style=Optimised  visibilities=8  version=20211007
  Shift1 : DSPBAPrim/Shift  primtype=shift  nInputs=2  nOutputs=1  omode=Inherit via internal rule  otype=sfix(16)  scale=2^-15  rndmethod=Unbiased  factor=1  satmethod=Symmetric  shift_vec=[0 1 2 -1]  value=0  inPortNames=['a'; 'b';]  outPortNames=[' ']  dspbaimage=dspba_prim.svg  text=fprintf('a >> b');  style=Optimised  visibilities=8  version=20211007
  dout : Outport
  wires:
  SampleDelay2/1 -> Relational Operator/2
  Shift/1 -> SampleDelay1/1, Scope/3, dout/1
  RegField2/1 -> Scope/2, Shift1/2, Shift/2
  din/1 -> Scope/1, Shift/1, Shift1/1
  Relational Operator/1 -> Assertion/1
  Shift1/1 -> Scope/4, SampleDelay2/1
  SampleDelay1/1 -> Relational Operator/1

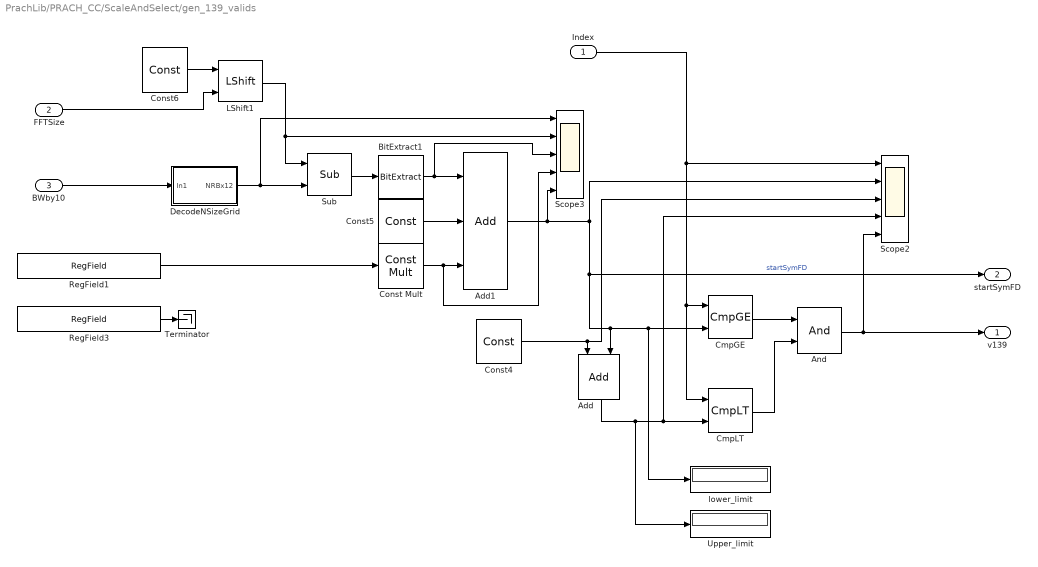
== system PrachLib/PRACH_CC/ScaleAndSelect/gen_139_valids ==
  Index : Inport
  FFTSize : Inport  Port=2
  BWby10 : Inport  Port=3
  Add : DSPBAPrim/Add  primtype=add  nInputs=evalAionMaskParam(gcb,'value',1)  nOutputs=1  omode=Inherit via internal rule with word growth  otype=sfix(16)  scale=2^-15  rndmethod=Unbiased  factor=1  satmethod=Symmetric  shift_vec=[0 1 2 -1]  value=2  inPortNames=[' '; ' ';]  outPortNames=[' ']  dspbaimage=dspba_prim.svg  text=fprintf('+');  style=Optimised  visibilities=1032+2^17+2^18+2^19  genFPC=off  floatRounding=correct  advOptions=[]  version=20211007
  Add1 : DSPBAPrim/Add  primtype=add  nInputs=evalAionMaskParam(gcb,'value',1)  nOutputs=1  omode=Specify via dialog  otype=ufix(log2(prach_short.Nfft))  scale=1  rndmethod=Unbiased  factor=1  satmethod=Symmetric  shift_vec=[0 1 2 -1]  value=3  inPortNames=[' '; ' ';]  outPortNames=[' ']  dspbaimage=dspba_prim.svg  text=fprintf('+');  style=Optimised  visibilities=1032+2^17+2^18+2^19  genFPC=off  floatRounding=correct  advOptions=[]  version=20211007
  And : DSPBAPrim/And  primtype=and  nInputs=2  nOutputs=1  omode=Inherit via internal rule  otype=sfix(16)  scale=2^-15  rndmethod=Unbiased  factor=1  satmethod=Symmetric  shift_vec=[0 1 2 -1]  value=0  inPortNames=[' '; ' '; ' '; ' '; ' '; ' '; ' '; ' '; ' '; ' '; ' '; ' '; ' '; ' '; ' '; ' '; ]  outPortNames=[' ']  dspbaimage=dspba_prim.svg  text=fprintf('&');  style=Optimised  visibilities=8+2  version=20211007
  BitExtract1 : DSPBAPrim/BitExtract  primtype=bitextract  nInputs=1  nOutputs=1  omode=Inherit via internal rule  otype=ufix(1)  scale=1  rndmethod=Unbiased  factor=1  satmethod=Symmetric  shift_vec=[0 1 2 -1]  value=1  inPortNames=[' '; ' ';]  outPortNames=[' ']  dspbaimage=dspba_prim.svg  text=fprintf('..%d', value);  style=Optimised  visibilities=8+1024  version=20211007
  CmpGE : DSPBAPrim/CmpGE  primtype=cmpgte  nInputs=2  nOutputs=1  omode=boolean  otype=sfix(16)  scale=2^-15  rndmethod=Unbiased  factor=1  satmethod=Symmetric  shift_vec=[0 1 2 -1]  value=0  inPortNames=['a'; 'b';]  outPortNames=[' ']  dspbaimage=dspba_prim.svg  text=fprintf('a>=b');  style=Optimised  visibilities=0  advOptions=[]  version=20211007
  CmpLT : DSPBAPrim/CmpLT  primtype=cmplt  nInputs=2  nOutputs=1  omode=boolean  otype=sfix(16)  scale=2^-15  rndmethod=Unbiased  factor=1  satmethod=Symmetric  shift_vec=[0 1 2 -1]  value=0  inPortNames=['a'; 'b';]  outPortNames=[' ']  dspbaimage=dspba_prim.svg  text=fprintf('a<b');  style=Optimised  visibilities=0  advOptions=[]  version=20211007
  Const Mult : DSPBAPrim/Const Mult  primtype=constmult  nInputs=1  nOutputs=1  omode=Inherit via internal rule  otype=sfix(16)  scale=2^-15  rndmethod=Unbiased  factor=1  satmethod=Symmetric  shift_vec=[0 1 2 -1]  value=12  inPortNames=[' '; ' ';]  outPortNames=[' ']  dspbaimage=dspba_prim.svg  text=fprintf('cx');  style=Optimised  visibilities=8+2^10+2^17+2^18  floatRounding=correct  advOptions=[]  version=20211007
  Const4 : DSPBAPrim/Const  primtype=const  nInputs=0  nOutputs=1  omode=Inherit via internal rule  otype=sfix(16)  scale=2^-15  rndmethod=Unbiased  factor=1  satmethod=Symmetric  shift_vec=[0 1 2 -1]  value=139  inPortNames=['+'; '+';]  outPortNames=[' ']  dspbaimage=dspba_prim.svg  text=fprintf('%s', num2str(value));  style=Optimised  visibilities=8 + 1024  floatPrecision=float32_m23  warnSaturation=on  version=20211007  SampleTime=inf
  Const5 : DSPBAPrim/Const  primtype=const  nInputs=0  nOutputs=1  omode=Inherit via internal rule  otype=sfix(16)  scale=2^-15  rndmethod=Unbiased  factor=1  satmethod=Symmetric  shift_vec=[0 1 2 -1]  value=3  inPortNames=['+'; '+';]  outPortNames=[' ']  dspbaimage=dspba_prim.svg  text=fprintf('%s', num2str(value));  style=Optimised  visibilities=8 + 1024  floatPrecision=float32_m23  warnSaturation=on  version=20211007  SampleTime=inf
  Const6 : DSPBAPrim/Const  primtype=const  nInputs=0  nOutputs=1  omode=Inherit via internal rule  otype=sfix(16)  scale=2^-15  rndmethod=Unbiased  factor=1  satmethod=Symmetric  shift_vec=[0 1 2 -1]  value=1  inPortNames=['+'; '+';]  outPortNames=[' ']  dspbaimage=dspba_prim.svg  text=fprintf('%s', num2str(value));  style=Optimised  visibilities=8 + 1024  floatPrecision=float32_m23  warnSaturation=on  version=20211007  SampleTime=inf
  DecodeNSizeGrid : Subsystem
  LShift1 : DSPBAPrim/LShift  primtype=lshift  nInputs=2  nOutputs=1  omode=Specify via dialog  otype=ufix(log2(prach_short.Nfft))  scale=1  rndmethod=Unbiased  factor=1  satmethod=Symmetric  shift_vec=[0 1 2 -1]  value=0  inPortNames=['a'; 'b';]  outPortNames=[' ']  dspbaimage=dspba_prim.svg  text=fprintf('a << b');  style=Optimised  visibilities=8  version=20211007
  RegField1 : DSPBAModelBus/RegField  reg_name=PRACH_regs(InstanceNumber).PRACH_RB_offset_addr  reg_rwmode=Read/Write  reg_msb=log2(prach_short.Nfft)-1  reg_lsb=0  reg_mode=Specify via dialog  reg_type=ufix(log2(prach_short.Nfft))  reg_scale=1  reg_init=PRACH_regs(InstanceNumber).PRACH_RB_offset  reg_desc=PRACH_regs(InstanceNumber).PRACH_RB_offset_string  reg_modal=off  reg_desc0=0  reg_desc1=0  reg_desc2=0  reg_desc3=0  reg_desc4=0  reg_desc5=0  reg_desc6=0  reg_desc7=0  reg_addr=13  SampleTime=-1  version=20090407
  RegField3 : DSPBAModelBus/RegField  reg_name=PRACH_regs(InstanceNumber).PRACH_freq_index_addr  reg_rwmode=Read/Write  reg_msb=log2(prach_short.Nfft)-1  reg_lsb=0  reg_mode=Specify via dialog  reg_type=ufix(log2(prach_short.Nfft))  reg_scale=1  reg_init=PRACH_regs(InstanceNumber).PRACH_freq_index  reg_desc=PRACH_regs(InstanceNumber).PRACH_freq_index_string  reg_modal=off  reg_desc0=0  reg_desc1=0  reg_desc2=0  reg_desc3=0  reg_desc4=0  reg_desc5=0  reg_desc6=0  reg_desc7=0  reg_addr=14  SampleTime=-1  version=20090407
  Scope2 : Scope  NumInputPorts=5
  Scope3 : Scope  NumInputPorts=5
  Sub : DSPBAPrim/Sub  primtype=sub  nInputs=2  nOutputs=1  omode=Specify via dialog  otype=ufix(log2(prach_short.Nfft))  scale=1  rndmethod=Unbiased  factor=1  satmethod=Symmetric  shift_vec=[0 1 2 -1]  value=0  inPortNames=['+'; '-';]  outPortNames=[' ']  dspbaimage=dspba_prim.svg  text=fprintf('-');  style=Optimised  visibilities=8+2^17+2^18  floatRounding=correct  advOptions=[]  version=20211007
  Terminator : Terminator
  Upper_limit : Display
  lower_limit : Display
  v139 : Outport
  startSymFD : Outport  Port=2
  wires:
  Index/1 -> Scope2/1, CmpGE/1, CmpLT/1
  Add1/1 -> Scope3/5, Scope2/2, startSymFD/1, Add/2, lower_limit/1, CmpGE/2  "startSymFD"
  Const Mult/1 -> Scope3/4, Add1/3
  Const4/1 -> Scope2/3, Add/1
  RegField3/1 -> Terminator/1
  Sub/1 -> BitExtract1/1
  BitExtract1/1 -> Scope3/3, Add1/1
  And/1 -> v139/1, Scope2/5
  Const6/1 -> LShift1/1
  CmpLT/1 -> And/2
  CmpGE/1 -> And/1
  Add/1 -> Upper_limit/1, Scope2/4, CmpLT/2
  Const5/1 -> Add1/2
  LShift1/1 -> Sub/1, Scope3/2
  DecodeNSizeGrid/1(NRBx12) -> Scope3/1, Sub/2
  BWby10/1 -> DecodeNSizeGrid/1(In1)
  RegField1/1 -> Const Mult/1
  FFTSize/1 -> LShift1/2

== system PrachLib/Stream2BlockConv/RdAddrGen/latch_0L ==
  e : Inport
  d : Inport  Port=2
  Mux : DSPBAPrim/Mux  primtype=mux  nInputs=evalAionMaskParam(gcb,'value',1)+1  nOutputs=1  omode=Inherit via internal rule  otype=sfix(16)  scale=2^-15  rndmethod=Unbiased  factor=1  satmethod=Symmetric  shift_vec=[0 1 2 -1]  value=2  inPortNames=['s'; 'd0'; 'd1'; 'd2'; 'd3'; 'd4'; 'd5'; 'd6'; 'd7'; 'd8'; 'd9';]  outPortNames=[' ']  dspbaimage=dspba_prim_tall.svg  text=fprintf('%s', primtype);  style=Optimised  visibilities=1032  version=20211007
  SameDT : DSPBAControl/SameDT
  SampleDelay : DSPBAPrim/SampleDelay  primtype=sampdelay  nInputs=1  nOutputs=1  omode=boolean  otype=uint(16)  scale=2^-0  rndmethod=Unbiased  factor=1  satmethod=Symmetric  shift_vec=[0 1 2 -1]  floatPrecision=float32_m23  value=1  inPortNames=[' '; ' ';]  outPortNames=[' ']  dspbaimage=dspba_prim.svg  text=dpoly(1, eye(1,value+1), 'z')  style=Optimised  visibilities=8 + 1024  flexible=off  slackgroup=0  augmented=0  version=20211007  advOptions=[]
  q : Outport
  wires:
  d/1 -> Mux/3, SameDT/1
  e/1 -> Mux/1
  SampleDelay/1 -> Mux/2, q/1
  Mux/1 -> SampleDelay/1, SameDT/2

== system PrachLib/Stream2BlockConv/WrCtrl/bitrev ==
  NatIn : Inport
  FFTSize : Inport  Port=2
  BitReverse : DSPBAPrim/BitReverse  primtype=bitrev  nInputs=1  nOutputs=1  omode=Inherit via internal rule  otype=sfix(16)  scale=2^-15  rndmethod=Unbiased  factor=1  satmethod=Symmetric  shift_vec=[0 1 2 -1]  value=0  inPortNames=[' '; ' ';]  outPortNames=[' ']  dspbaimage=dspba_prim.svg  text=fprintf('rev');  style=Optimised  visibilities=0  version=20211007
  Const2 : DSPBAPrim/Const  primtype=const  nInputs=0  nOutputs=1  omode=Inherit via internal rule  otype=sfix(16)  scale=2^-15  rndmethod=Unbiased  factor=1  satmethod=Symmetric  shift_vec=[0 1 2 -1]  value=log2(NFftMax)  inPortNames=['+'; '+';]  outPortNames=[' ']  dspbaimage=dspba_prim.svg  text=fprintf('%s', num2str(value));  style=Optimised  visibilities=8 + 1024  floatPrecision=float32_m23  warnSaturation=on  version=20211007  SampleTime=inf
  Shift : DSPBAPrim/Shift  primtype=shift  nInputs=2  nOutputs=1  omode=Specify via dialog  otype=ufix(ceil(log2(prach_short.Nfft)))  scale=1  rndmethod=Unbiased  factor=1  satmethod=Symmetric  shift_vec=[0 1 2 -1]  value=0  inPortNames=['a'; 'b';]  outPortNames=[' ']  dspbaimage=dspba_prim.svg  text=fprintf('a >> b');  style=Optimised  visibilities=8  version=20211007
  Sub : DSPBAPrim/Sub  primtype=sub  nInputs=2  nOutputs=1  omode=Specify via dialog  otype=ufix(4)  scale=1  rndmethod=Unbiased  factor=1  satmethod=Symmetric  shift_vec=[0 1 2 -1]  value=0  inPortNames=['+'; '-';]  outPortNames=[' ']  dspbaimage=dspba_prim.svg  text=fprintf('-');  style=Optimised  visibilities=8+2^17+2^18  floatRounding=correct  advOptions=[]  version=20211007
  WriteScope2 : Scope  NumInputPorts=4
  BitReversedOut : Outport
  NatOut : Outport  Port=2
  wires:
  Shift/1 -> BitReversedOut/1, WriteScope2/1
  Sub/1 -> WriteScope2/4, Shift/2
  Const2/1 -> Sub/1
  FFTSize/1 -> Sub/2
  NatIn/1 -> BitReverse/1, WriteScope2/3, NatOut/1
  BitReverse/1 -> Shift/1, WriteScope2/2
